simulink model "fuzzy_PID_control"  (R2021a)
settings: Solver=VariableStepAuto  StartTime=0.0  StopTime=100  RelTol=1e-3
libraries: fuzblock x1
settings Model: Creator=hty  LastModifiedBy=hty

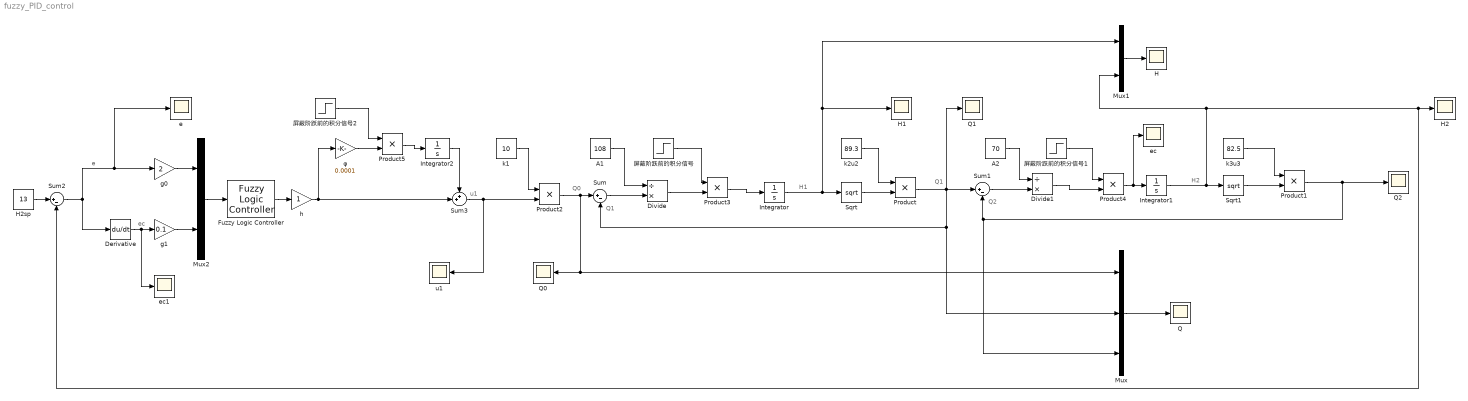
== system fuzzy_PID_control ==
  note: ec
  note: Q1
  note: e
  note: H2
  note: Q2
  note: H1
  note: Q1
  note: Q0
  note: u1
  A1 : Constant  Value=108
  A2 : Constant  Value=70
  Derivative : Derivative
  Divide : Product  Inputs=/*
  Divide1 : Product  Inputs=/*
  Fuzzy Logic Controller : fuzblock/Fuzzy Logic  Controller  FIS='fuzzy_rules.fis'  OutputSampleNumber=101  DataType=double  FuzzifiedInputs=off  RuleFiringStrengths=off  RuleOutputs=off  AggregatedOutputs=off  SimulateUsing=Interpreted execution  OutOfRangeInputValueMessage=warning  NoRuleFiredMessage=warning  EmptyOutputFuzzySetMessage=warning
  H : Scope
  H1 : Scope
  H2 : Scope
  H2sp : Constant  Value=13
  Integrator : Integrator  InitialCondition=10
  Integrator1 : Integrator  InitialCondition=13
  Integrator2 : Integrator  LimitOutput=on  UpperSaturationLimit=0.1  LowerSaturationLimit=-0.1
  Mux : Mux  Inputs=3
  Mux1 : Mux  Inputs=2
  Mux2 : Mux  Inputs=2
  Product{,1..5} (6 alike) : Product
  Q{,0..2} (4 alike) : Scope
  Sqrt : Sqrt  SaturateOnIntegerOverflow=on
  Sqrt1 : Sqrt  SaturateOnIntegerOverflow=on
  Sum : Sum  Inputs=|+-
  Sum1 : Sum  Inputs=|+-
  Sum2 : Sum  Inputs=|+-
  Sum3 : Sum  Inputs=++|
  e : Scope
  ec : Scope
  ec1 : Scope
  g0 : Gain  Gain=2
  g1 : Gain  Gain=0.1
  h : Gain
  k1 : Constant  Value=10
  k2u2 : Constant  Value=89.3
  k3u3 : Constant  Value=82.5
  u1 : Scope
  φ : Gain  Gain=0.0001
  屏蔽阶跃前的积分信号 : Step  Time=5  SampleTime=0
  屏蔽阶跃前的积分信号1 : Step  Time=5  SampleTime=0
  屏蔽阶跃前的积分信号2 : Step  Time=5  SampleTime=0
  wires:
  Sqrt1/1 -> Product1/2
  Integrator/1 -> Mux1/1, H1/1, Sqrt/1
  k3u3/1 -> Product1/1
  Product2/1 -> Mux/1, Q0/1, Sum/1
  Derivative/1 -> ec1/1, g1/1
  Product/1 -> Mux/2, Sum/2, Q1/1, Sum1/1
  Divide/1 -> Product3/2
  Product1/1 -> Mux/3, Sum1/2, Q2/1
  Integrator1/1 -> Sum2/2, H2/1, Mux1/2, Sqrt1/1
  Mux1/1 -> H/1
  g0/1 -> Mux2/1
  Fuzzy Logic Controller/1 -> h/1
  屏蔽阶跃前的积分信号/1 -> Product3/1
  g1/1 -> Mux2/2
  Mux/1 -> Q/1
  A2/1 -> Divide1/1
  Product4/1 -> ec/1, Integrator1/1
  Divide1/1 -> Product4/2
  Sum1/1 -> Divide1/2
  屏蔽阶跃前的积分信号1/1 -> Product4/1
  Sum2/1 -> e/1, g0/1, Derivative/1
  Mux2/1 -> Fuzzy Logic Controller/1
  k1/1 -> Product2/1
  Product3/1 -> Integrator/1
  H2sp/1 -> Sum2/1
  Sqrt/1 -> Product/2
  Sum/1 -> Divide/2
  A1/1 -> Divide/1
  k2u2/1 -> Product/1
  h/1 -> φ/1, Sum3/2
  Sum3/1 -> u1/1, Product2/2
  φ/1 -> Product5/2
  Product5/1 -> Integrator2/1
  屏蔽阶跃前的积分信号2/1 -> Product5/1
  Integrator2/1 -> Sum3/1
